simulink model "PowerWindows"  (R2020b)
settings: Solver=VariableStepAuto  StartTime=0.0  StopTime=10.0  RelTol=1e-3
settings Model: Creator=99003778  LastModifiedBy=99003778

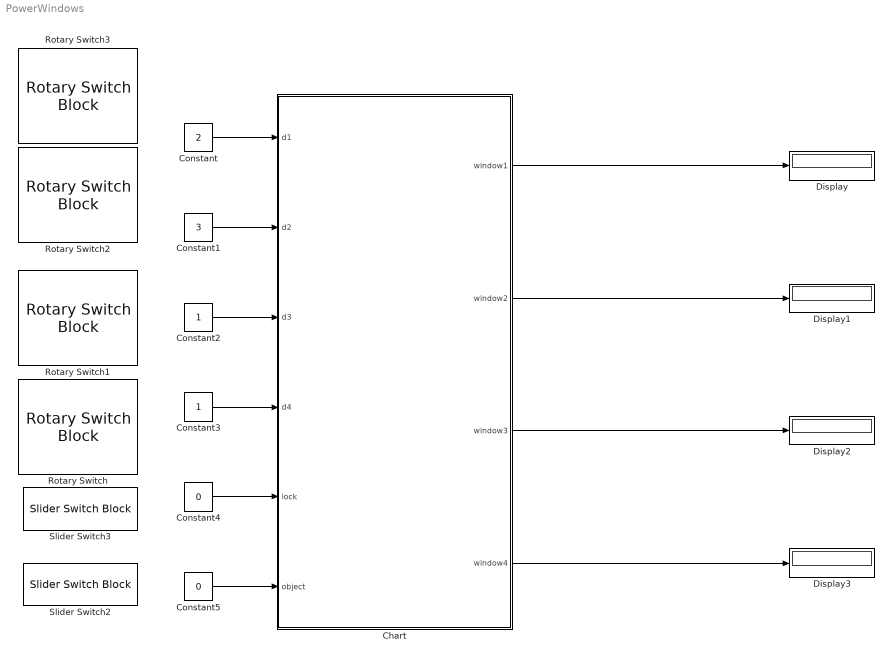
== system PowerWindows ==
  Chart : Stateflow chart  TreatAsAtomicUnit=on
  Constant : Constant  Value=2
  Constant1 : Constant  Value=3
  Constant2 : Constant
  Constant3 : Constant
  Constant4 : Constant  Value=0
  Constant5 : Constant  Value=0
  Display{,1..3} (4 alike) : Display
  Rotary Switch{,1..3} (4 alike) : RotarySwitchBlock
      settings: Values={{'Off', 'Low', 'Medium', 'High'}, [0 1 2 3]}
  Slider Switch2 : SliderSwitchBlock
      settings: Values={{'Off', 'On'}, [0 1]}
  Slider Switch3 : SliderSwitchBlock
      settings: Values={{'Off', 'On'}, [0 1]}
  wires:
  Constant/1 -> Chart/1(d1)
  Constant1/1 -> Chart/2(d2)
  Constant2/1 -> Chart/3(d3)
  Constant3/1 -> Chart/4(d4)
  Constant4/1 -> Chart/5(lock)
  Constant5/1 -> Chart/6(object)
  Chart/1(window1) -> Display/1
  Chart/2(window2) -> Display1/1
  Chart/3(window3) -> Display2/1
  Chart/4(window4) -> Display3/1

== stateflow chart PowerWindows/Chart ==
  state window1_1
    entry:
    window1=25;
  note: [d2== 1 &&lock== 1 ]
  state window2_1
    entry:
    window1=25;
  state window1_2
    entry:
    window1=50;
  state window2_2
    entry:
    window1=50;
  state default
    entry:
    window1=0;
    window2=0;
    window3=0;
    window4=0;
  state window1_3
    entry:
    window1=75;
  state window2_3
    entry:
    window1=75;
  state window1_4
    entry:
    window1=100;
  state window2_4
    entry:
    window1=100;
  state window3_1
    entry:
    window1=25;
  state window4_1
    entry:
    window1=25;
  state window3_2
    entry:
    window1=50;
  state window4_2
    entry:
    window1=50;
  state window3_3
    entry:
    window1=75;
  state window4_3
    entry:
    window1=75;
  state window3_4
    entry:
    window1=100;
  state window4_4
    entry:
    window1=100;
  (junction 93) -> window2_1 [order 1] : [d2==1&&lock==1]
  (junction 93) -> window2_2 [order 2] : [d2==1&&lock==1]
  window1_1 -> (junction 93) [order 4] : [d2==1&&lock==1]
  (junction 93) -> window2_3 [order 3] : [d2==1&&lock==1]
  (junction 93) -> window2_4 [order 4] : [d2==1&&lock==1]
  window1_2 -> (junction 93) [order 4] : [d2==1&&lock==1]
  window1_3 -> (junction 93) [order 4]
  window1_4 -> (junction 93) [order 3] : [d2==1&&lock==1]
  (junction 132) -> window1_1 [order 4] : [d1==1&&lock==1]
  default -> window1_1 [order 1] : [d1==1&&lock==1]
  window2_1 -> (junction 123) [order 4] : [d3==1&&lock==1]
  window2_1 -> default [order 2] : [d2==1&&lock==0]
  window1_1 -> default [order 1] : [d1==0&&lock==1]
  window1_1 -> (junction 32) [order 3] : [object==1]
  default -> window2_1 [order 3] : [d2==1&&lock==1]
  window1_1 -> window1_2 [order 2] : [d1==2&&lock==1]
  window1_2 -> window1_1 [order 1] : [d1==1&&lock==1]
  window2_1 -> window2_2 [order 1] : [d2==2&&lock==1]
  window2_2 -> window2_1 [order 1] : [d2==1&&lock==1]
  window2_1 -> (junction 38) [order 3] : [object==1]
  (default) -> default
  window2_2 -> (junction 123) [order 4] : [d3==1&&lock==1]
  window1_2 -> (junction 32) [order 3] : [object==1]
  (junction 132) -> window1_2 [order 3] : [d1==1&&lock==1]
  window1_2 -> window1_3 [order 2] : [d1==3&&lock==1]
  window1_3 -> window1_2 [order 1] : [d1==2&&lock==1]
  window2_2 -> window2_3 [order 2] : [d2==3&&lock==1]
  window2_3 -> window2_2 [order 1] : [d2==2&&lock==1]
  window2_2 -> (junction 38) [order 3] : [object==1]
  window1_3 -> (junction 32) [order 3] : [object==1]
  (junction 132) -> window1_3 [order 2] : [d1==1&&lock==1]
  (junction 32) -> default
  window2_3 -> (junction 38) [order 3] : [object==1]
  (junction 38) -> default
  window1_4 -> (junction 32) [order 2] : [object==1]
  window2_4 -> (junction 38) [order 2] : [object==1]
  window2_3 -> (junction 123) [order 4] : [d3==1&&lock==1]
  window1_3 -> window1_4 [order 2] : [d1==4&&lock==1]
  window1_4 -> window1_3 [order 1] : [d1==3&&lock==1]
  window2_3 -> window2_4 [order 2] : [d2==4&&lock==1]
  window2_4 -> window2_3 [order 1] : [d2==3&&lock==1]
  (junction 132) -> window1_4 [order 1] : [d1==1&&lock==1]
  window2_4 -> (junction 123) [order 3] : [d3==1&&lock==1]
  window4_1 -> (junction 132) [order 4] : [d1==1&&lock==1]
  window4_2 -> (junction 132) [order 4] : [d1==1&&lock==1]
  window4_4 -> (junction 132) [order 3] : [d1==1&&lock==1]
  window4_3 -> (junction 132) [order 4] : [d1==1&&lock==1]
  (junction 123) -> window3_3 [order 3] : [d3==1&&lock==1]
  (junction 123) -> window3_1 [order 1] : [d3==1&&lock==1]
  (junction 123) -> window3_4 [order 4] : [d3==1&&lock==1]
  (junction 123) -> window3_2 [order 2] : [d3==1&&lock==1]
  window3_1 -> default [order 2] : [d3==0&&lock==1]
  window4_1 -> default [order 2] : [d4==0&&lock==1]
  default -> window3_1 [order 2] : [d3==1&&lock==1]
  default -> window4_1 [order 4] : [d4==1&&lock==1]
  window3_1 -> (junction 79) [order 3] : [object==1]
  window3_1 -> (junction 92) [order 4] : [d4==1&&lock==1]
  window4_1 -> (junction 80) [order 3] : [object==1]
  window3_1 -> window3_2 [order 1] : [d3==2&&lock==1]
  window3_2 -> window3_1 [order 1] : [d3==1&&lock==1]
  window4_1 -> window4_2 [order 1] : [d4==2&&lock==1]
  window4_2 -> window4_1 [order 1] : [d4==1&&lock==1]
  window4_2 -> (junction 80) [order 3] : [object==1]
  window3_2 -> (junction 79) [order 3] : [object==1]
  window3_2 -> window3_3 [order 2] : [d3==3&&lock==1]
  window3_3 -> window3_2 [order 1] : [d3==2&&lock==1]
  window3_2 -> (junction 92) [order 4] : [d4==1&&lock==1]
  window4_2 -> window4_3 [order 2] : [d4==3&&lock==1]
  window4_3 -> window4_2 [order 1] : [d4==2&&lock==1]
  window3_3 -> (junction 92) [order 4] : [d4==1&&lock==1]
  (junction 80) -> default
  window4_3 -> (junction 80) [order 3] : [object==1]
  window4_4 -> (junction 80) [order 2] : [object==1]
  window3_3 -> (junction 79) [order 3] : [object==1]
  (junction 79) -> default
  window3_3 -> window3_4 [order 2] : [d3==4&&lock==1]
  window3_4 -> window3_3 [order 1] : [d3==3&&lock==1]
  window3_4 -> (junction 79) [order 2] : [object==1]
  window4_3 -> window4_4 [order 2] : [d4==4&&lock==1]
  window4_4 -> window4_3 [order 1] : [d4==3&&lock==1]
  (junction 92) -> window4_4 [order 1] : [d4==1&&lock==1]
  window3_4 -> (junction 92) [order 3] : [d4==1&&lock==1]
  (junction 92) -> window4_4 [order 4] : [d4==1&&lock==1]
  (junction 92) -> window4_4 [order 2] : [d4==1&&lock==1]
  (junction 92) -> window4_4 [order 3] : [d4==1&&lock==1]
  data: d1 input; d2 input; d3 input; d4 input; lock input; object input; window1 output; window2 output; window3 output; window4 output
